simulink model "TK_Lineal_1"  (Simulink 6.1)
settings: Solver=ode45  StartTime=0.0  StopTime=10.0  RelTol=1e-3
settings Model: LastModifiedBy=Usuario
settings OptimizationCC: BlockReduction=off  BooleanDataType=off
settings HardwareCC: TargetUnknown=on

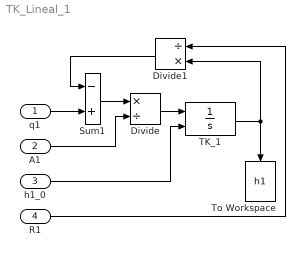
== system TK_Lineal_1 ==
  q1 : Inport  Port=1  LatchInput=off
  A1 : Inport  Port=2  LatchInput=off
  h1_0 : Inport  Port=3  LatchInput=off
  R1 : Inport  Port=4  LatchInput=off
  Divide : Product  Inputs=*/  OutScaling=2^-10
  Divide1 : Product  Orientation=left  Inputs=/*  OutScaling=2^-10
  Sum1 : Sum  Inputs=-+  SaturateOnIntegerOverflow=on  InputSameDT=on
  TK_1 : Integrator  InitialConditionSource=external
  To Workspace : ToWorkspace  VariableName=h1  SampleTime=-1  SaveFormat=Structure
      settings: Orientation=down
  wires:
  TK_1/1 -> To Workspace/1, Divide1/2
  Sum1/1 -> Divide/1
  Divide1/1 -> Sum1/1
  q1/1 -> Sum1/2
  A1/1 -> Divide/2
  Divide/1 -> TK_1/1
  h1_0/1 -> TK_1/2
  R1/1 -> Divide1/1
